simulink model "AAI_Version1"  (R2022a)
settings: Solver=FixedStepAuto  StartTime=0.0  StopTime=10.0  FixedStep=1e-3  RelTol=1e-3  EnableMultiTasking=on
undefined symbols (not defined in the file): D0, D10, D11, D12, D13, D2, D4, D5, D6, D7, D8, D9, PTA0, PTA2, PTB23, PTB9, PTC16, PTC2, PTC3, PTC4, PTD0, PTD1, PTD2, PTD3
libraries: frdmk64flib x12
settings Model: ExtModeTrigDuration=5  Creator=ethan  LastModifiedBy=ethan
settings OptimizationCC: EnhancedBackFolding=on  PassReuseOutputArgsAs=Individual arguments  ZeroExternalMemoryAtStartup=off  ZeroInternalMemoryAtStartup=off  MaxStackSize=64  OptimizeBlockOrder=speed  DifferentSizesBufferReuse=on  OptimizationCustomize=off  EfficientTunableParamExpr=on
settings DebuggingCC: ParameterTunabilityLossMsg=error
settings HardwareCC: ProdBitPerPointer=32  ProdBitPerSizeT=32  ProdBitPerPtrDiffT=32  ProdLargestAtomicInteger=Long  ProdLargestAtomicFloat=Double  ProdWordSize=32  ProdHWDeviceType=ARM Compatible->ARM Cortex
settings SFSimCC: MATLABDynamicMemAlloc=off
settings RTWCC: SystemTargetFile=ert.tlc  HardwareBoard=NXP FRDM-K64F  TLCOptions="-aInlineSetEventsForThisBaseRateFcn=TLC_FALSE -aSuppressMultiTaskScheduler=TLC_FALSE  -aRateBasedStepFcn=0"  TemplateMakefile=ert_default_tmf  Toolchain=GNU Tools for ARM Embedded Processors
settings CodeAppCC: ForceParamTrailComments=on  IgnoreCustomStorageClasses=off  OperatorAnnotations=on  SimulinkDataObjDesc=on  SFDataObjDesc=on  InsertBlockDesc=on
settings ERTTargetCC: ExtModeTransport=4  ExtModeMexFile=sendToCommService

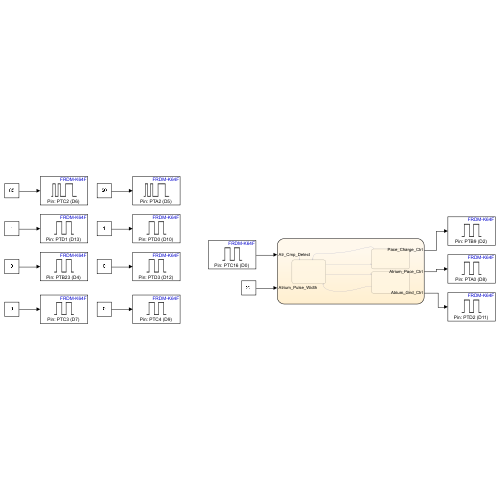
[thumbnail: Simulink's stored preview of the top-level diagram]
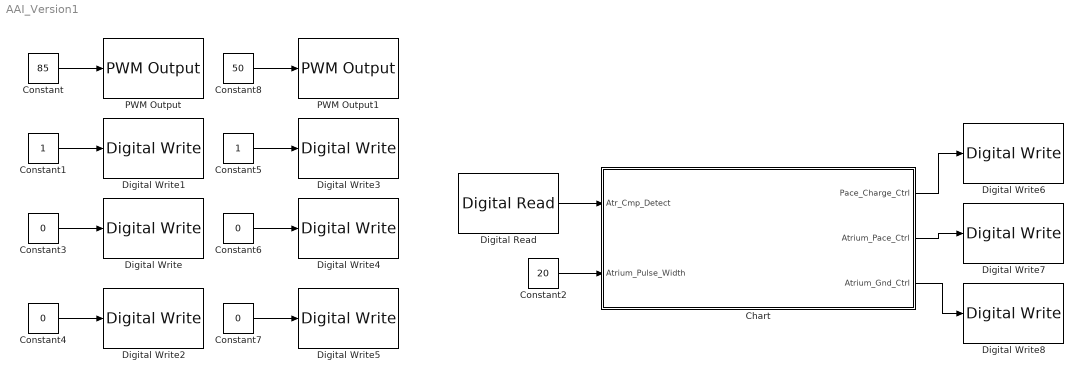
== system AAI_Version1 ==
  Chart : Stateflow chart  TreatAsAtomicUnit=on
  Constant : Constant  Value=85  OutDataTypeStr=int8
  Constant1 : Constant
  Constant2 : Constant  Value=20
  Constant{3..4,6..7} (4 alike) : Constant  Value=0
  Constant5 : Constant
  Constant8 : Constant  Value=50  OutDataTypeStr=int8
  Digital Read : frdmk64flib/Digital Read  Whichpin=PTC16 (D0)  SampleTime=-1
  Digital Write : frdmk64flib/Digital Write  Whichpin=PTB23 (D4)
  Digital Write1 : frdmk64flib/Digital Write  Whichpin=PTD1 (D13)
  Digital Write2 : frdmk64flib/Digital Write  Whichpin=PTC3 (D7)
  Digital Write3 : frdmk64flib/Digital Write  Whichpin=PTD0 (D10)
  Digital Write4 : frdmk64flib/Digital Write  Whichpin=PTD3 (D12)
  Digital Write5 : frdmk64flib/Digital Write  Whichpin=PTC4 (D9)
  Digital Write6 : frdmk64flib/Digital Write  Whichpin=PTB9 (D2)
  Digital Write7 : frdmk64flib/Digital Write  Whichpin=PTA0 (D8)
  Digital Write8 : frdmk64flib/Digital Write  Whichpin=PTD2 (D11)
  PWM Output : frdmk64flib/PWM Output  Whichpin=PTC2 (D6)  InitialFrequency=2000  InitialDutyCycle=0
  PWM Output1 : frdmk64flib/PWM Output  Whichpin=PTA2 (D5)  InitialFrequency=2000  InitialDutyCycle=0
  wires:
  Digital Read/1 -> Chart/1(Atr_Cmp_Detect)
  Constant/1 -> PWM Output/1
  Constant1/1 -> Digital Write1/1
  Constant2/1 -> Chart/2(Atrium_Pulse_Width)
  Constant3/1 -> Digital Write/1
  Constant4/1 -> Digital Write2/1
  Constant5/1 -> Digital Write3/1
  Constant6/1 -> Digital Write4/1
  Constant7/1 -> Digital Write5/1
  Chart/1(Pace_Charge_Ctrl) -> Digital Write6/1
  Chart/3(Atrium_Gnd_Ctrl) -> Digital Write8/1
  Chart/2(Atrium_Pace_Ctrl) -> Digital Write7/1
  Constant8/1 -> PWM Output1/1

== stateflow chart AAI_Version1/Chart ==
  state Inhibit
    entry:
    Pace_Charge_Ctrl = false;
    Atrium_Pace_Ctrl = true;
    Atrium_Gnd_Ctrl = true;
  state Signal_Search
    entry:
    Atrium_Pace_Ctrl = false;
    Atrium_Gnd_Ctrl = true;
    Pace_Charge_Ctrl = true;
  state Pace
    entry:
    Pace_Charge_Ctrl = false;
    Atrium_Pace_Ctrl = true;
    Atrium_Gnd_Ctrl = false;
  Inhibit -> Signal_Search : after(Atrium_Pulse_Width,msec)
  (default) -> Signal_Search
  Signal_Search -> Inhibit [order 1] : [Atr_Cmp_Detect == true]
  Signal_Search -> Pace [order 2] : [Atr_Cmp_Detect == false]
  Pace -> Signal_Search : after(Atrium_Pulse_Width,msec)
  data: Atr_Cmp_Detect input; Atrium_Cmp_Detect local; Atrium_Pulse_Width input; Pace_Charge_Ctrl output; Atrium_Pace_Ctrl output; Atrium_Gnd_Ctrl output
